simulink model "servo_model_verification"  (R2015a)
settings: Solver=ode8  StartTime=0.0  StopTime=60  FixedStep=0.01  RelTol=1e-3
StartFcn:
  | servo_param
values from neighbouring files (symbols this model uses):
  max_voltage = 13.3    [experiment1.mat]    (also in experiment2.mat; experiment3.mat; experiment4.mat; friction_ident.mat)
undefined symbols (not defined in the file or in its folder): sigbuilder_block
settings Model: Creator=Student  LastModifiedBy=Student

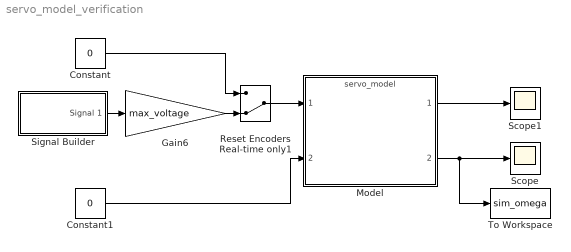
== system servo_model_verification ==
  Constant : Constant  Value=0
  Constant1 : Constant  Value=0
  Gain6 : Gain  Gain=max_voltage
  Model : ModelReference  ModelNameDialog=servo_model  SimulationMode=Normal  ModelReferenceVersion=1.27  CopyOfModelName=servo_model  DefaultDataLogging=on
  Reset Encoders Real-time only1 : ManualSwitch  CurrentSetting=0
  Scope : Scope
  Scope1 : Scope
  Signal Builder : Subsystem  Tag=STV Subsys  LoadFcn=sigbuilder_block('load');  StartFcn=sigbuilder_block('start');  StopFcn=sigbuilder_block('stop');  ClipboardFcn=sigbuilder_block('clipboard');  mask(Sigbuilder block){}
      mask help: Simulink:masks:SigbuilderBlock_MD
      mask init:
      | if ~strcmp(get_param(bdroot(gcbh),'SimulationStatus'),'stopped') tuvar = sigbuilder_block('maskInit'); end
      settings: CopyFcn=sigbuilder_block('copy');  DeleteFcn=sigbuilder_block('delete');  ModelCloseFcn=sigbuilder_block('modelClose');  PreSaveFcn=sigbuilder_block('preSave');  PauseFcn=sigbuilder_block('pause');  ContinueFcn=sigbuilder_block('continue');  NameChangeFcn=sigbuilder_block('namechange');  OpenFcn=sigbuilder_block('open',[437.6 199.2 550.4 400 ]);  CloseFcn=sigbuilder_block('close');
      mask Display: plot(0, 0, 100, 100,[2, 2, 32, 32, 2], [68, 8, 8, 68, 68],[32, 2], [38, 38], [32, 19, 2],[53, 60, 44], [32, 17, 17, 2],[16, 16, 31, 31]);txt = getActiveGroup(gcbh);text(2, 100, txt,'verticalAlignment', 'top');
  To Workspace : ToWorkspace  VariableName=sim_omega  SampleTime=-1
  wires:
  Signal Builder/1(Signal 1) -> Gain6/1
  Gain6/1 -> Reset Encoders Real-time only1/2
  Constant/1 -> Reset Encoders Real-time only1/1
  Reset Encoders Real-time only1/1 -> Model/1
  Model/2 -> Scope/1, To Workspace/1
  Model/1 -> Scope1/1
  Constant1/1 -> Model/2

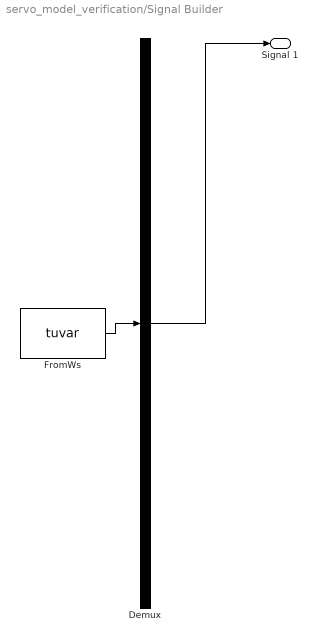
== system servo_model_verification/Signal Builder ==
  Demux : Demux  Tag=STV Demux  Outputs=1
  FromWs : FromWorkspace  Tag=STV FromWs  VariableName=tuvar  SampleTime=0
      SigBuilderData=|
      | common.afterFinalStr = 'Extrapolate'
      | common.sampleTime = 0
      | dataSet.timeRange = [0 50]
      | dataSet.name = 'Group 1'
      | sbobj.Groups.Name = 'Group 1'
      | sbobj.Groups.Signals.Name = 'Signal 1'
      | sbobj.Groups.Signals.XData = [0 0.1 0.1 10 10 20.1 20.1 30.1 30.1 39.9 39.9 50]
      | sbobj.Groups.Signals.YData = [0 0 0.2 0.2 0.405 0.405 0.604 0.604 0.8 0.8 0.995 0.995]
      | sbobj.Groups.TimeRange = [0 50]
  Signal 1 : Outport  Tag=STV Outport
  wires:
  Demux/1 -> Signal 1/1
  FromWs/1 -> Demux/1
